simulink model "mut_discrete_time_integrator"  (R2020b)
settings: Solver=VariableStepAuto  StartTime=0.0  StopTime=10.0  RelTol=1e-3
values from neighbouring files (symbols this model uses):
  parSampTime = 0.01    [dd_discrete_time_integrator.sldd]
libraries: vhit_control_library x1
settings Model: DataDictionary=dd_discrete_time_integrator.sldd  EnableAccessToBaseWorkspace=off  Creator=CAV2OFO  LastModifiedBy=CAV2OFO

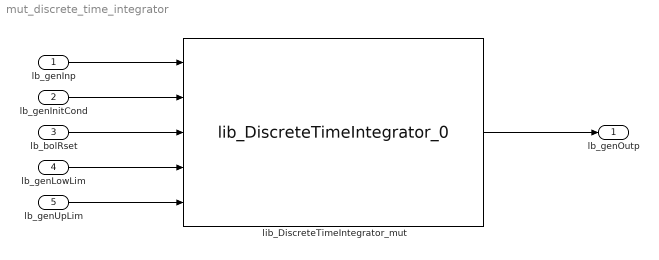
== system mut_discrete_time_integrator ==
  lb_genInp : Inport  OutDataTypeStr=parInpDataType  SampleTime=double(parSampTime)
  lb_genInitCond : Inport  Port=2  OutDataTypeStr=parOutpDataType  SampleTime=double(parSampTime)
  lb_bolRset : Inport  Port=3  OutDataTypeStr=boolean  SampleTime=double(parSampTime)
  lb_genLowLim : Inport  Port=4  OutDataTypeStr=parOutpDataType  SampleTime=double(parSampTime)
  lb_genUpLim : Inport  Port=5  OutDataTypeStr=parOutpDataType  SampleTime=double(parSampTime)
  lib_DiscreteTimeIntegrator_mut : vhit_control_library/lib_DiscreteTimeIntegrator_0  lb_parSampTime=parSampTime  lb_parIntgGain=parIntgGain  lb_parAccmDataType=parAccmDataType  lb_parOutpDataType=Inherit: Inherit via back propagation  lb_parSatFlag=off
  lb_genOutp : Outport  OutDataTypeStr=parOutpDataType  SampleTime=double(parSampTime)
  wires:
  lb_genLowLim/1 -> lib_DiscreteTimeIntegrator_mut/4
  lb_bolRset/1 -> lib_DiscreteTimeIntegrator_mut/3
  lb_genUpLim/1 -> lib_DiscreteTimeIntegrator_mut/5
  lb_genInp/1 -> lib_DiscreteTimeIntegrator_mut/1
  lib_DiscreteTimeIntegrator_mut/1 -> lb_genOutp/1
  lb_genInitCond/1 -> lib_DiscreteTimeIntegrator_mut/2
